simulink model "pratica2_2_ac"  (R2021a)
settings: Solver=VariableStepAuto  StartTime=0.0  StopTime=10.0  RelTol=1e-3
settings Model: Creator=ribeiro  LastModifiedBy=ribeiro

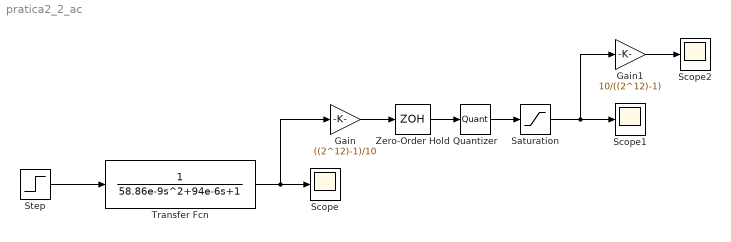
== system pratica2_2_ac ==
  Gain : Gain  Gain=((2^12)-1)/10
  Gain1 : Gain  Gain=10/((2^12)-1)
  Quantizer : Quantizer  QuantizationInterval=1/((2^12)-1)
  Saturation : Saturate  UpperLimit=(2^12)-1  LowerLimit=0
  Scope : Scope
  Scope1 : Scope
  Scope2 : Scope
  Step : Step  After=10  SampleTime=0
  Transfer Fcn : TransferFcn  Numerator=1  Denominator=[58.86e-9 94e-6 1]
  Zero-Order Hold : ZeroOrderHold  SampleTime=1/100
  wires:
  Transfer Fcn/1 -> Gain/1, Scope/1
  Zero-Order Hold/1 -> Quantizer/1
  Quantizer/1 -> Saturation/1
  Saturation/1 -> Gain1/1, Scope1/1
  Gain/1 -> Zero-Order Hold/1
  Gain1/1 -> Scope2/1
  Step/1 -> Transfer Fcn/1
